simulink model "Task08_Model_Delay"  (R2026a)
settings: Solver=VariableStepAuto
settings Model: Creator=Tommy  LastModifiedBy=Tommy

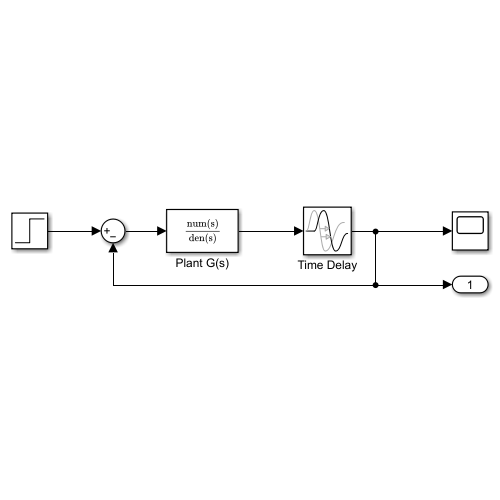
[thumbnail: Simulink's stored preview of the top-level diagram]
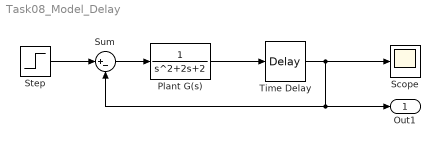
== system Task08_Model_Delay ==
  Plant G(s) : TransferFcn  Denominator=[1 2 2]
  Scope : Scope
  Step : Step  SampleTime=0
  Sum : Sum  Inputs=|+-
  Time Delay : TransportDelay
  Out1 : Outport
  wires:
  Step/1 -> Sum/1
  Sum/1 -> Plant G(s)/1
  Plant G(s)/1 -> Time Delay/1
  Time Delay/1 -> Sum/2, Out1/1, Scope/1
